simulink model "CoupledTanksRp"  (Simulink 7.3)
settings: Solver=ode45  StartTime=0.0  StopTime=60  RelTol=1e-3
InitFcn:
  | g = 9.81; %gravitational constant
  | r = 980; %density of water
  | 
  | %% S-function
  | % showVR = 0;
  | % h1_init = 0; %initial conditions
  | % h2_init = 0; %initial conditions
libraries: vrlib x6
CloseFcn:
  | vrclose all;
  | clear figureVR worldVR;
settings Model: Creator=H  LastModifiedBy=Ivo
settings DataIOCC: ReturnWorkspaceOutputs=off
settings OptimizationCC: InitFltsAndDblsToZero=on
settings DebuggingCC: SaveWithParameterizedLinksMsg=none  SignalResolutionControl=TryResolveAllWithWarning
settings GRTTargetCC: TargetFcnLib=ansi_tfl_tmw.mat

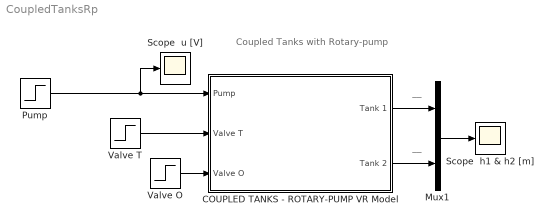
== system CoupledTanksRp ==
  note: Coupled Tanks
      | with Rotary-pump
  note: __
  note: __
  COUPLED TANKS - ROTARY-PUMP VR Model : Subsystem  mask(Coupled Tanks with Rotary Pump){showVR=off, h1_0=0, h2_0=0}
      mask prompts: showVR "Show VirtualWorld?"; h1_0 "Initial fluid level in the tank 1   h1(0)  [cm]"; h2_0 "Initial fluid  level in the tank 2   h2 (0) [cm]"
      mask help: Coupled Tanks with Rotary Pump - Virtual Reality
      mask init:
      | clear figureVR worldVR;
      | showVR = 1;
      mask Help:
      | Couple Tankswith Rotary Pump - Virtual Reality. <br><br>
      | 
      | 
      | This is a model of the Coupled Tanks, which consists of a rotary-pump, two tanks (left and right), inflow and outflow pipes and  transfer and output valves. The left tank is filled with the fluid by the rotary-pump and the fluid drains away to the right tank through the transfer valve and from the right tank drains away through the output valve. The system input is the voltage of the motor of the rotary-pump and the system outputs are the levels of the fluid in the tanks. The dynamics of the rotary-pump motor is neglected. <br><br>
      | 
      | 
      | In the mask of the model, it can be set:
      | <ul>
      | <li>Initial fluid level in the left tank</li>
      | <li>Initial fluid level in the right tank.</li>
      | </ul><br><br>
      | 
      | 
      | Copyright: 2007, Jan Vana, Jirka Roubal, Petr Husek.
      mask CallbackString:
      | if strcmp('off',get_param(gcb,'showVR'))
      |     vrclose all;
      | else
      |     if exist('figureVR')==0
      |         figureVR = vrfigure;
      |     end
      |     if exist('worldVR')==0
      |         worldVR = vrworld('CoupledTanks_VR.WRL');
      |     end
      | 	if isvalid(figureVR)==0
      |         open(worldVR);
      |         figureVR = vrfigure(worldVR,[650 80 550 350]);
      | 	end
      | end||
      mask Display:
      | image(imread('CoupledTanks_Image.jpg'));
      | port_label ('input',1,'u')
      | port_label ('input',2,'Valve T')
      | port_label ('input',3,'Valve O')
      | port_label ('output',1,'h1')
      | port_label ('output',2,'h2')
  Mux1 : Mux  Inputs=2
  Pump : Step  Time=0  After=10  SampleTime=0
  Scope  h1 & h2 [m] : Scope
      settings: TimeRange=60  YMin=2.77556e-17  YMax=0.7  SaveName=ty  MaxDataPoints=5000000
  Scope  u [V] : Scope
      settings: TimeRange=600  YMin=0  YMax=7  SaveName=tu  MaxDataPoints=5000000
  Valve O : Step  Time=0  After=0.1  SampleTime=0
  Valve T : Step  Time=0  After=0.1  SampleTime=0
  wires:
  COUPLED TANKS - ROTARY-PUMP VR Model/1(Tank 1) -> Mux1/1
  Mux1/1 -> Scope  h1 & h2 [m]/1
  Valve T/1 -> COUPLED TANKS - ROTARY-PUMP VR Model/2(Valve T)
  Valve O/1 -> COUPLED TANKS - ROTARY-PUMP VR Model/3(Valve O)
  Pump/1 -> Scope  u [V]/1, COUPLED TANKS - ROTARY-PUMP VR Model/1(Pump)
  COUPLED TANKS - ROTARY-PUMP VR Model/2(Tank 2) -> Mux1/2

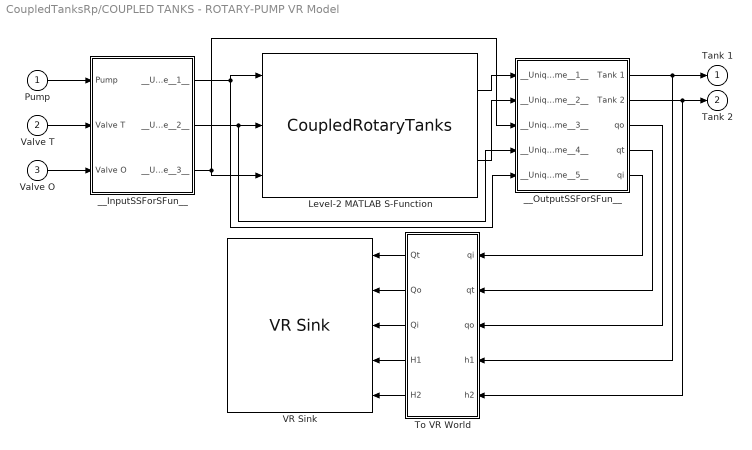
== system CoupledTanksRp/COUPLED TANKS - ROTARY-PUMP VR Model ==
  Pump : Inport
  Valve T : Inport  Port=2
  Valve O : Inport  Port=3
  Level-2 MATLAB S-Function : M-S-Function  FunctionName=CoupledRotaryTanks  Parameters=h1_0 h2_0  mask{h1_0=h1_0, h2_0=h2_0}
      mask Display:
      | port_label('output', 1, 'Tank 1')
      | port_label('output', 2, 'Tank 2')
      | port_label('input', 1, 'Pump')
      | port_label('input', 2, 'Valve T')
      | port_label('input', 3, 'Valve O')
  To VR World : Subsystem
  VR Sink : vrlib/VR Sink  InstantiateOnLoad=on  SampleTime=0.1  ViewEnable=on  RemoteChange=off  RemoteView=on  FieldsWritten=pumpOut.rotation.4.1.double#pumpOut2.rotation.4.1.double#pump.rotation.4.1.double#water1.scale.3.1.double#water2.scale.3.1.double  WorldFileName=CoupledTanks_VR.WRL  AutoView=off  VideoDimensions=[]
  __InputSSForSFun__ : Subsystem
      settings: PermitHierarchicalResolution=ParametersOnly
  __OutputSSForSFun__ : Subsystem
      settings: PermitHierarchicalResolution=ParametersOnly
  Tank 1 : Outport  OutDataTypeStr=double  PortDimensions=1  SampleTime=[-1 0]  DataType=double
  Tank 2 : Outport  Port=2  OutDataTypeStr=double  PortDimensions=1  SampleTime=[-1 0]  DataType=double
  wires:
  __OutputSSForSFun__/3(qo) -> To VR World/3(qo)
  __OutputSSForSFun__/4(qt) -> To VR World/2(qt)
  __OutputSSForSFun__/5(qi) -> To VR World/1(qi)
  To VR World/5(H2) -> VR Sink/5
  To VR World/4(H1) -> VR Sink/4
  To VR World/3(Qi) -> VR Sink/3
  To VR World/2(Qo) -> VR Sink/2
  To VR World/1(Qt) -> VR Sink/1
  __OutputSSForSFun__/2(Tank 2) -> To VR World/5(h2), Tank 2/1
  __OutputSSForSFun__/1(Tank 1) -> Tank 1/1, To VR World/4(h1)
  Level-2 MATLAB S-Function/2 -> __OutputSSForSFun__/2(__UniqueInportName__2__)
  Level-2 MATLAB S-Function/1 -> __OutputSSForSFun__/1(__UniqueInportName__1__)
  __InputSSForSFun__/3(__UniqueOutportName__3__) -> __OutputSSForSFun__/3(__UniqueInportName__3__), Level-2 MATLAB S-Function/3
  __InputSSForSFun__/2(__UniqueOutportName__2__) -> __OutputSSForSFun__/4(__UniqueInportName__4__), Level-2 MATLAB S-Function/2
  __InputSSForSFun__/1(__UniqueOutportName__1__) -> __OutputSSForSFun__/5(__UniqueInportName__5__), Level-2 MATLAB S-Function/1
  Valve O/1 -> __InputSSForSFun__/3(Valve O)
  Valve T/1 -> __InputSSForSFun__/2(Valve T)
  Pump/1 -> __InputSSForSFun__/1(Pump)

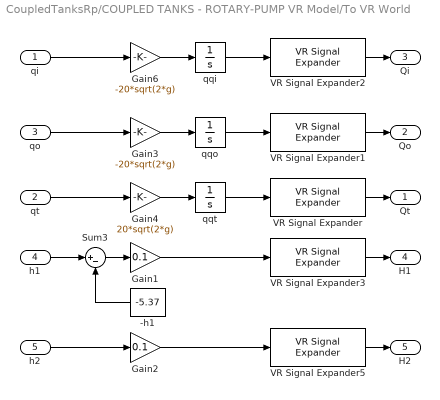
== system CoupledTanksRp/COUPLED TANKS - ROTARY-PUMP VR Model/To VR World ==
  qi : Inport
  qt : Inport  Port=2
  qo : Inport  Port=3
  h1 : Inport  Port=4
  h2 : Inport  Port=5
  -h1 : Constant  Value=-5.37
  Gain1 : Gain  Gain=0.1
  Gain2 : Gain  Gain=0.1
  Gain3 : Gain  Gain=-20*sqrt(2*g)
  Gain4 : Gain  Gain=20*sqrt(2*g)
  Gain6 : Gain  Gain=-20*sqrt(2*g)
  Sum3 : Sum  Inputs=|+-
  VR Signal Expander : vrlib/VR Signal Expander  outwidth=4  outidx=[4]
  VR Signal Expander1 : vrlib/VR Signal Expander  outwidth=4  outidx=[4]
  VR Signal Expander2 : vrlib/VR Signal Expander  outwidth=4  outidx=[4]
  VR Signal Expander3 : vrlib/VR Signal Expander  outwidth=3  outidx=[2]
  VR Signal Expander5 : vrlib/VR Signal Expander  outwidth=3  outidx=[2]
  qqi : Integrator
  qqo : Integrator
  qqt : Integrator
  Qt : Outport
  Qo : Outport  Port=2
  Qi : Outport  Port=3
  H1 : Outport  Port=4
  H2 : Outport  Port=5
  wires:
  qi/1 -> Gain6/1
  h1/1 -> Sum3/1
  Sum3/1 -> Gain1/1
  -h1/1 -> Sum3/2
  qqo/1 -> VR Signal Expander1/1
  qqt/1 -> VR Signal Expander/1
  Gain4/1 -> qqt/1
  Gain6/1 -> qqi/1
  Gain3/1 -> qqo/1
  qt/1 -> Gain4/1
  qo/1 -> Gain3/1
  Gain2/1 -> VR Signal Expander5/1
  Gain1/1 -> VR Signal Expander3/1
  VR Signal Expander5/1 -> H2/1
  VR Signal Expander3/1 -> H1/1
  VR Signal Expander2/1 -> Qi/1
  VR Signal Expander1/1 -> Qo/1
  VR Signal Expander/1 -> Qt/1
  h2/1 -> Gain2/1
  qqi/1 -> VR Signal Expander2/1

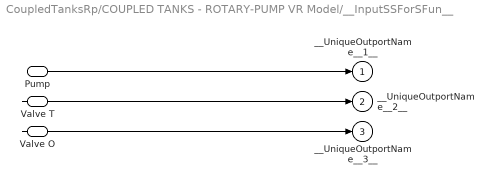
== system CoupledTanksRp/COUPLED TANKS - ROTARY-PUMP VR Model/__InputSSForSFun__ ==
  Pump : Inport
  Valve T : Inport  Port=2
  Valve O : Inport  Port=3
  __UniqueOutportName__1__ : Outport
  __UniqueOutportName__2__ : Outport  Port=2
  __UniqueOutportName__3__ : Outport  Port=3
  wires:
  Valve O/1 -> __UniqueOutportName__3__/1
  Valve T/1 -> __UniqueOutportName__2__/1
  Pump/1 -> __UniqueOutportName__1__/1

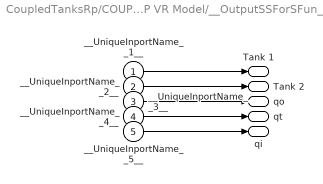
== system CoupledTanksRp/COUPLED TANKS - ROTARY-PUMP VR Model/__OutputSSForSFun__ ==
  __UniqueInportName__1__ : Inport
  __UniqueInportName__2__ : Inport  Port=2
  __UniqueInportName__3__ : Inport  Port=3
  __UniqueInportName__4__ : Inport  Port=4
  __UniqueInportName__5__ : Inport  Port=5
  Tank 1 : Outport  OutDataTypeStr=double  PortDimensions=1  SampleTime=[-1 0]  DataType=double
  Tank 2 : Outport  Port=2  OutDataTypeStr=double  PortDimensions=1  SampleTime=[-1 0]  DataType=double
  qo : Outport  Port=3  OutDataTypeStr=double  PortDimensions=1  SampleTime=[-1 0]  DataType=double
  qt : Outport  Port=4  OutDataTypeStr=double  PortDimensions=1  SampleTime=[-1 0]  DataType=double
  qi : Outport  Port=5  OutDataTypeStr=double  PortDimensions=1  SampleTime=[-1 0]  DataType=double
  wires:
  __UniqueInportName__5__/1 -> qi/1
  __UniqueInportName__4__/1 -> qt/1
  __UniqueInportName__3__/1 -> qo/1
  __UniqueInportName__2__/1 -> Tank 2/1
  __UniqueInportName__1__/1 -> Tank 1/1
